simulink model "GPS_IMU_KF"  (R2013b)
settings: Solver=FixedStepDiscrete  StartTime=0.0  StopTime=10.0  FixedStep=0.1  RelTol=1e-3
settings Model: Creator=echo  LastModifiedBy=建云
settings RTWCC: SystemTargetFile=NIVeriStand.tlc  TemplateMakefile=NIVeriStand_vc.tmf  Description=NI VeriStand Real-Time Target for Release 2007b or later  ProcessScript=NIVeriStand_make_rtw_hook
settings STFCustomTargetCC: GeneratePreprocessorConditionals=Disable all  MatFileLogging=on  MATLABClassNameForMDSCustomization=Simulink.SoftwareTarget.TargetSpecificTriggerConfigurationBase  SystemTargetFile=NIVeriStand.tlc

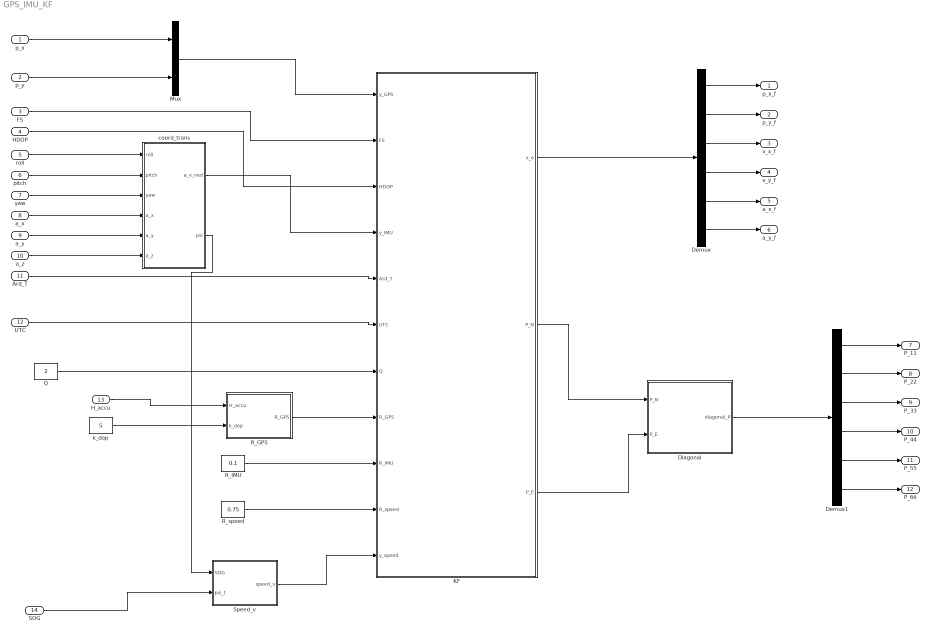
== system GPS_IMU_KF ==
  p_x : Inport
  p_y : Inport  Port=2
  FS : Inport  Port=3
  HDOP : Inport  Port=4
  roll : Inport  Port=5
  pitch : Inport  Port=6
  yaw : Inport  Port=7
  a_x : Inport  Port=8
  a_y : Inport  Port=9
  a_z : Inport  Port=10
  Ard_T : Inport  Port=11
  UTC : Inport  Port=12
  H_accu : Inport  Port=13
  SOG : Inport  Port=14
  Demux : Demux  Outputs=6
  Demux1 : Demux  Outputs=6
  Diagonal : MATLAB Function  TreatAsAtomicUnit=on
  KF : MATLAB Function  TreatAsAtomicUnit=on
  Mux : Mux  Inputs=2
  Q : Constant  Value=2
  R_GPS : MATLAB Function  TreatAsAtomicUnit=on
  R_IMU : Constant  Value=0.1
  R_speed : Constant  Value=0.75
  Speed_v : MATLAB Function  TreatAsAtomicUnit=on
  coord_trans : MATLAB Function  TreatAsAtomicUnit=on
  k_dop : Constant  Value=5
  p_x_f : Outport
  p_y_f : Outport  Port=2
  v_x_f : Outport  Port=3
  v_y_f : Outport  Port=4
  a_x_f : Outport  Port=5
  a_y_f : Outport  Port=6
  P_11 : Outport  Port=7
  P_22 : Outport  Port=8
  P_33 : Outport  Port=9
  P_44 : Outport  Port=10
  P_55 : Outport  Port=11
  P_66 : Outport  Port=12
  wires:
  p_x/1 -> Mux/1
  p_y/1 -> Mux/2
  roll/1 -> coord_trans/1(roll)
  pitch/1 -> coord_trans/2(pitch)
  yaw/1 -> coord_trans/3(yaw)
  a_y/1 -> coord_trans/5(a_y)
  a_z/1 -> coord_trans/6(a_z)
  coord_trans/1(a_v_ned) -> KF/4(y_IMU)
  Ard_T/1 -> KF/5(Ard_T)
  UTC/1 -> KF/6(UTC)
  Q/1 -> KF/7(Q)
  R_IMU/1 -> KF/9(R_IMU)
  KF/1(x_e) -> Demux/1
  KF/2(P_N) -> Diagonal/1(P_N)
  FS/1 -> KF/2(FS)
  HDOP/1 -> KF/3(HDOP)
  Demux/1 -> p_x_f/1
  Demux/2 -> p_y_f/1
  Mux/1 -> KF/1(y_GPS)
  Diagonal/1(diagonal_P) -> Demux1/1
  Demux1/1 -> P_11/1
  Demux1/2 -> P_22/1
  Demux1/3 -> P_33/1
  Demux1/4 -> P_44/1
  Demux1/5 -> P_55/1
  Demux1/6 -> P_66/1
  Demux/3 -> v_x_f/1
  Demux/4 -> v_y_f/1
  Demux/5 -> a_x_f/1
  Demux/6 -> a_y_f/1
  H_accu/1 -> R_GPS/1(H_accu)
  k_dop/1 -> R_GPS/2(k_dop)
  R_GPS/1(R_GPS) -> KF/8(R_GPS)
  coord_trans/2(psi) -> Speed_v/1(SOG)
  SOG/1 -> Speed_v/2(psi_t)
  Speed_v/1(speed_v) -> KF/11(y_speed)
  KF/3(P_E) -> Diagonal/2(P_E)
  a_x/1 -> coord_trans/4(a_x)
  R_speed/1 -> KF/10(R_speed)

== matlab function GPS_IMU_KF/coord_trans ==
  data: roll input; a_v_ned output; pitch input; yaw input; a_x input; a_y input; a_z input; psi output
function [a_v_ned,psi] = coord_Trans(roll, pitch, yaw, a_x, a_y, a_z)
mag_decl = 10;
phi = roll*pi/180;
theta = pitch*pi/180;
yaw_t = yaw + mag_decl;
psi = yaw_t*pi/180;
a_v = [a_x, a_y, a_z]';
J_trans = [cos(psi)*cos(theta), -sin(psi)*cos(phi)+cos(psi)*sin(theta)*sin(phi), sin(psi)*sin(phi)+cos(psi)*cos(phi)*sin(theta);
    sin(psi)*cos(theta), cos(psi)*cos(phi)+sin(phi)*sin(theta)*sin(psi), -cos(psi)*sin(phi)+sin(theta)*sin(psi)*cos(phi);
    -sin(theta), cos(theta)*sin(phi), cos(theta)*cos(phi)];
tmp = J_trans*a_v;
a_v_ned = tmp(1:2);

== matlab function GPS_IMU_KF/KF ==
  data: y_GPS input; FS input; HDOP input; y_IMU input; Ard_T input; x_e output; UTC input; Q input; R_GPS input; R_IMU input; R_speed input; P_N output; P_E output; y_speed input
function [x_e, P_N, P_E] = KF_1(y_GPS, FS, HDOP, y_IMU, Ard_T, UTC, Q, R_GPS,R_IMU, R_speed, y_speed)

persistent velLimit
if isempty(velLimit)
    velLimit = 4;
end
persistent accLimit
if isempty(accLimit)
    accLimit = 2;
end

gps_valid_flag = 1;

persistent Ard_T_old
if isempty(Ard_T_old)
    Ard_T_old = Ard_T;
end
T = (Ard_T - Ard_T_old)/1000;
Ard_T_old = Ard_T;

persistent UTC_old
if isempty(UTC_old)
    UTC_old = UTC;
end

persistent x_e_1_N P_1_N
if isempty(x_e_1_N)
    x_e_1_N = [y_GPS(1);0;0];
end
if isempty(P_1_N)
    P_1_N = 1000*eye(3);
end
persistent x_e_1_E P_1_E
if isempty(x_e_1_E)
    x_e_1_E = [y_GPS(2);0;0];
end
if isempty(P_1_E)
    P_1_E = eye(3);
end

%% Dead Reckoning
persistent k_gps
if isempty(k_gps)
    k_gps = 0;
end
persistent GPS_p_x_old GPS_p_y_old
if isempty(GPS_p_x_old)
    GPS_p_x_old = y_GPS(1);
end
if isempty(GPS_p_y_old)
    GPS_p_y_old = y_GPS(2);
end
persistent interval
if isempty(interval)
    interval = 0.1;
end
if UTC == UTC_old || FS == 0 
    gps_valid_flag = 0;
end
UTC_old = UTC;

%% remove bad points
persistent y_IMU_old
if isempty(y_IMU_old)
    y_IMU_old = y_IMU;
end
if y_IMU'*y_IMU > 1
    y_IMU = y_IMU_old;
end
%% select observation vector
if gps_valid_flag == 0
    k_gps = k_gps + 1;
    p_x_dr = GPS_p_x_old + y_speed(1)*interval*k_gps;
    p_y_dr = GPS_p_y_old + y_speed(2)*interval*k_gps;
    y_GPS_IMU_N = [p_x_dr; y_speed(1); y_IMU(1)]; 
    y_GPS_IMU_E = [p_y_dr; y_speed(2); y_IMU(2)];
else
    GPS_p_x_old = y_GPS(1);
    GPS_p_y_old = y_GPS(2);
    y_GPS_IMU_N = [y_GPS(1); y_speed(1); y_IMU(1)];
    y_GPS_IMU_E = [y_GPS(2); y_speed(2); y_IMU(2)];
end
%%
R_GPS = HDOP^2*R_GPS;
if gps_valid_flag == 1
    R_GPS = R_GPS*k_gps^2;
end

Phi = [eye(1), T*eye(1), T^2/2*eye(1);
       zeros(1), eye(1), T*eye(1);
       zeros(1), zeros(1), eye(1)]; % transfer matrix
Sigma = [T^3/6*ones(1,1);T^2/2*ones(1,1);T*ones(1,1)];
persistent H_GPS_IMU
if isempty(H_GPS_IMU)
    H_GPS_IMU = eye(3);
end
%% kf --north
R_GPS_IMU_N = [R_GPS(1,1),  0,  0;
              0,   R_speed,  0;
              0,   0,    R_IMU];
Q_N = Q;
%--------------- 1 step prediction ----------------
x_1_p_N = Phi*x_e_1_N;
P_1_p_N = Phi*P_1_N*Phi' + Sigma*Q_N*Sigma';
%--------------- innovation------------------
%GPS_IMU
epsilon_GPS_IMU_N = y_GPS_IMU_N - H_GPS_IMU*x_1_p_N;
Q_ep_GPS_IMU_N = H_GPS_IMU*P_1_p_N*H_GPS_IMU' + R_GPS_IMU_N;
K_GPS_IMU_N = P_1_p_N*H_GPS_IMU'*Q_ep_GPS_IMU_N^(-1);

%--------------------estimate------------------------
x_e_N = x_1_p_N + K_GPS_IMU_N*epsilon_GPS_IMU_N;
P_N = (eye(3) - K_GPS_IMU_N*H_GPS_IMU)*P_1_p_N;   

%% kf --east
R_GPS_IMU_E = [R_GPS(2,2),  0,  0;
              0,   R_speed,  0;
              0,   0,    R_IMU];
Q_E = Q;
%--------------- 1 step prediction ----------------
x_1_p_E = Phi*x_e_1_E;
P_1_p_E = Phi*P_1_E*Phi' + Sigma*Q_E*Sigma';
%--------------- innovation------------------
%GPS_IMU
epsilon_GPS_IMU_E = y_GPS_IMU_E - H_GPS_IMU*x_1_p_E;
Q_ep_GPS_IMU_E = H_GPS_IMU*P_1_p_E*H_GPS_IMU' + R_GPS_IMU_E;
K_GPS_IMU_E = P_1_p_E*H_GPS_IMU'*Q_ep_GPS_IMU_E^(-1);

%--------------------estimate------------------------
x_e_E = x_1_p_E + K_GPS_IMU_E*epsilon_GPS_IMU_E;
P_E = (eye(3) - K_GPS_IMU_E*H_GPS_IMU)*P_1_p_E;   

%%

if gps_valid_flag == 1
    k_gps = 0;
end
%% avoid steep change
persistent bad_point_count
if isempty(bad_point_count)
    bad_point_count = 0;
end
if (sqrt( (x_e_N(1)-x_e_1_N(1))^2 + (x_e_E(1)-x_e_1_E(1))^2 )/interval > velLimit)  %velocity > velLimit m/s
% if ((x_e_N(2)-x_e_1_N(2))/0.1 > accLimit || (x_e_E(2)-x_e_1_E(2))/0.1 > accLimit)
%     p_x_dr = x_e_1_N(1) + y_speed(1)*interval;
%     p_y_dr = x_e_1_E(1) + y_speed(2)*interval;
    x_e = [x_e_1_N(1);x_e_1_E(1);x_e_1_N(2);x_e_1_E(2);x_e_1_N(3);x_e_1_E(3)];
    bad_point_count = bad_point_count+1;
%     display(bad_point_count)
%     display(x_e_1)
%     display(T)
else
    x_e_1_N = x_e_N;
    P_1_N = P_N; 
    x_e_1_E = x_e_E;
    P_1_E = P_E; 
    x_e = [x_e_N(1);x_e_E(1);x_e_N(2);x_e_E(2);x_e_N(3);x_e_E(3)];
end
end

== matlab function GPS_IMU_KF/Diagonal ==
  data: P_N input; diagonal_P output; P_E input
function diagonal_P = Diagonal(P_N,P_E)
diagonal_P = zeros(6,1);
diagonal_P(1) = P_N(1);
diagonal_P(2) = P_E(1);
diagonal_P(3) = P_N(2);
diagonal_P(4) = P_E(2);
diagonal_P(5) = P_N(3);
diagonal_P(6) = P_E(3);

== matlab function GPS_IMU_KF/R_GPS ==
  data: H_accu input; R_GPS output; k_dop input
function R_GPS = R_GPS(H_accu, k_dop)
R_GPS = k_dop*[H_accu^2,0;0,H_accu^2];

== matlab function GPS_IMU_KF/Speed_v ==
  data: SOG input; speed_v output; psi_t input
function speed_v = speed_v(SOG, psi_t)
v_x = SOG*cos(psi_t); 
v_y = SOG*sin(psi_t);
speed_v = [v_x;v_y];
